simulink model "motorcdError"  (R2021a)
settings: Solver=VariableStepAuto  StartTime=0.0  StopTime=200.00  RelTol=1e-3
settings Model: Creator=User  LastModifiedBy=Bremdow

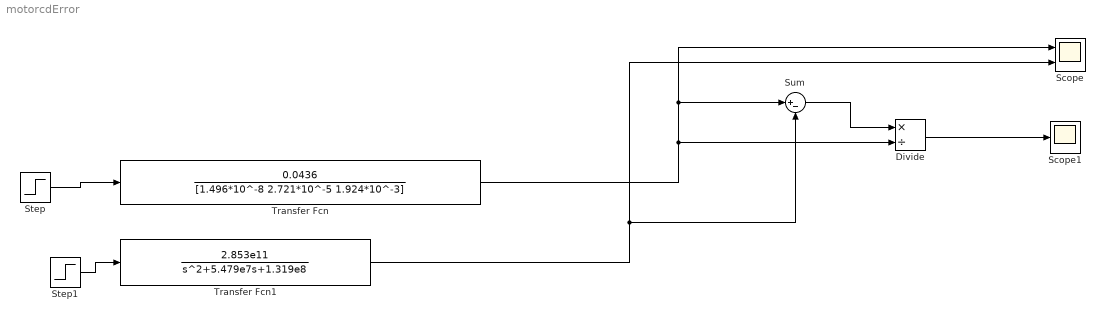
== system motorcdError ==
  Divide : Product  Inputs=*/
  Scope : Scope  NumInputPorts=2
  Scope1 : Scope
  Step : Step  Time=0  After=22  SampleTime=0
  Step1 : Step  Time=0  After=22  SampleTime=0
  Sum : Sum  Inputs=|+-
  Transfer Fcn : TransferFcn  Numerator=[0.0436]  Denominator=[1.496*10^-8 2.721*10^-5 1.924*10^-3]
  Transfer Fcn1 : TransferFcn  Numerator=[2.853e11]  Denominator=[1 5.479e7 1.319e8]
  wires:
  Step1/1 -> Transfer Fcn1/1
  Transfer Fcn/1 -> Divide/2, Scope/1, Sum/1
  Divide/1 -> Scope1/1
  Transfer Fcn1/1 -> Scope/2, Sum/2
  Sum/1 -> Divide/1
  Step/1 -> Transfer Fcn/1
